simulink model "kalman_filter"  (R2021a)
settings: Solver=FixedStepAuto  StartTime=0.0  StopTime=30-0.2  FixedStep=dt  RelTol=1e-3
values from neighbouring files (symbols this model uses):
  dt = 0.2    [kalman_filter_data.mat]
  m = 1000    [kalman_filter_data.mat]
  P = [1  0; 0  1]    [kalman_filter_data.mat]
  Q = [0.3  0; 0  0.1]    [kalman_filter_data.mat]
  r = 0.2    [kalman_filter_data.mat]
  R = 20    [kalman_filter_data.mat]
  x_hat = [0 0]    [kalman_filter_data.mat]
settings Model: Creator=Sıla The Magnificent  LastModifiedBy=Sıla The Magnificent

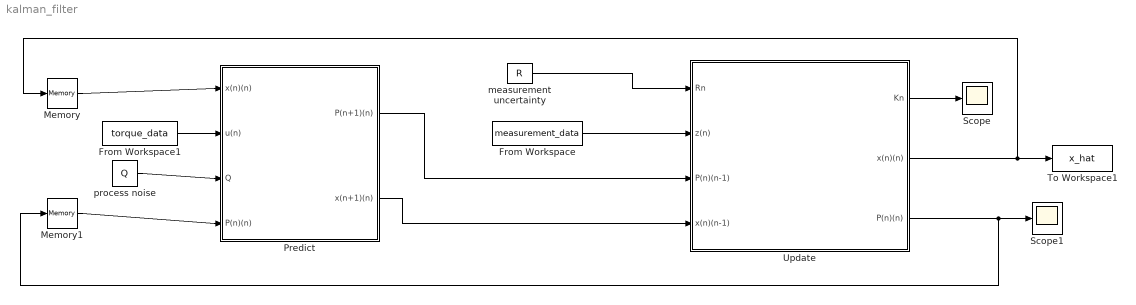
== system kalman_filter ==
  From Workspace : FromWorkspace  VariableName=measurement_data  SampleTime=dt
  From Workspace1 : FromWorkspace  VariableName=torque_data  SampleTime=dt
  Memory : Memory  InitialCondition=x_hat
  Memory1 : Memory  InitialCondition=P
  Predict : Subsystem
  Scope : Scope
  Scope1 : Scope
  To Workspace1 : ToWorkspace  VariableName=x_hat  SaveFormat=Timeseries  SampleTime=dt
  Update : Subsystem
  measurement uncertainty : Constant  Value=R  SampleTime=dt
  process noise : Constant  Value=Q  VectorParams1D=off  SampleTime=dt
  wires:
  From Workspace1/1 -> Predict/2(u(n))
  process noise/1 -> Predict/3(Q)
  measurement uncertainty/1 -> Update/1(Rn)
  From Workspace/1 -> Update/2(z(n))
  Predict/2(x(n+1)(n)) -> Update/4(x(n)(n-1))
  Predict/1(P(n+1)(n)) -> Update/3(P(n)(n-1))
  Update/1(Kn) -> Scope/1
  Update/2(x(n)(n)) -> Memory/1, To Workspace1/1
  Update/3(P(n)(n)) -> Scope1/1, Memory1/1
  Memory/1 -> Predict/1(x(n)(n))
  Memory1/1 -> Predict/4(P(n)(n))

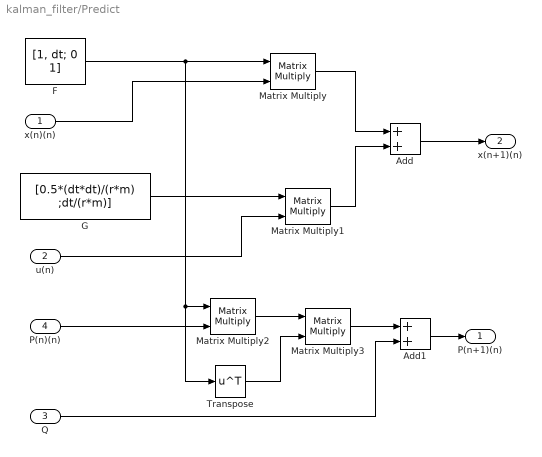
== system kalman_filter/Predict ==
  x(n)(n) : Inport
  u(n) : Inport  Port=2
  Q : Inport  Port=3
  P(n)(n) : Inport  Port=4
  Add : Sum
  Add1 : Sum
  F : Constant  Value=[1, dt; 0 1]  VectorParams1D=off  SampleTime=dt
  G : Constant  Value=[0.5*(dt*dt)/(r*m) ;dt/(r*m)]  VectorParams1D=off  SampleTime=dt
  Matrix Multiply{,1..3} (4 alike) : Product  Multiplication=Matrix(*)
  Transpose : Math  Operator=transpose  SaturateOnIntegerOverflow=on
  P(n+1)(n) : Outport
  x(n+1)(n) : Outport  Port=2
  wires:
  F/1 -> Matrix Multiply/1, Matrix Multiply2/1, Transpose/1
  x(n)(n)/1 -> Matrix Multiply/2
  Matrix Multiply/1 -> Add/1
  G/1 -> Matrix Multiply1/1
  u(n)/1 -> Matrix Multiply1/2
  Matrix Multiply1/1 -> Add/2
  Add/1 -> x(n+1)(n)/1
  P(n)(n)/1 -> Matrix Multiply2/2
  Matrix Multiply2/1 -> Matrix Multiply3/1
  Transpose/1 -> Matrix Multiply3/2
  Matrix Multiply3/1 -> Add1/1
  Q/1 -> Add1/2
  Add1/1 -> P(n+1)(n)/1

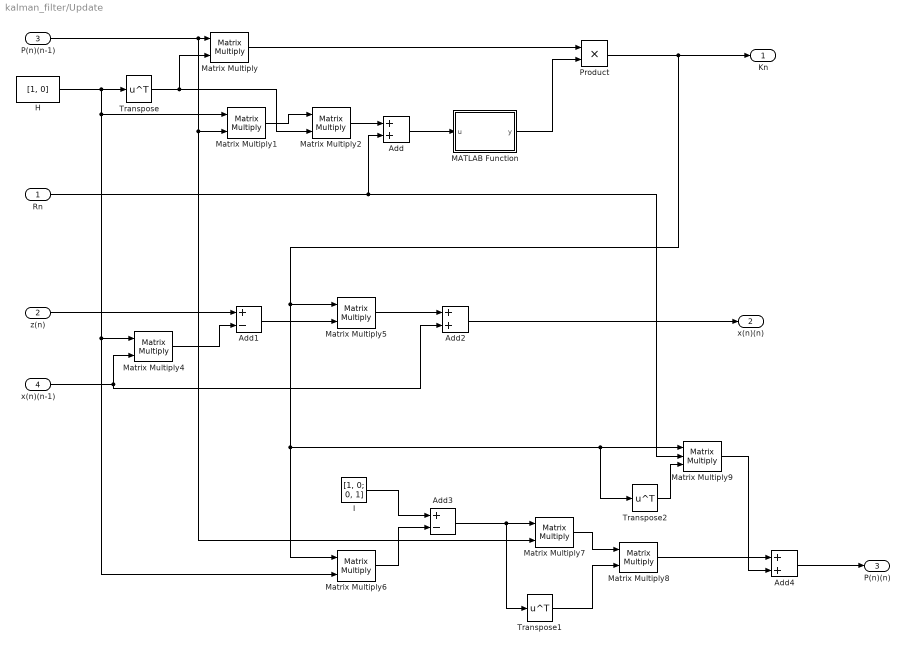
== system kalman_filter/Update ==
  Rn : Inport
  z(n) : Inport  Port=2
  P(n)(n-1) : Inport  Port=3
  x(n)(n-1) : Inport  Port=4
  Add : Sum
  Add1 : Sum  Inputs=+-
  Add2 : Sum
  Add3 : Sum  Inputs=+-
  Add4 : Sum
  H : Constant  Value=[1, 0]  VectorParams1D=off  SampleTime=dt
  I : Constant  Value=[1, 0; 0, 1]  VectorParams1D=off  SampleTime=dt
  MATLAB Function : MATLAB Function  TreatAsAtomicUnit=on
  Matrix Multiply{,1..2,4..8} (8 alike) : Product  Multiplication=Matrix(*)
  Matrix Multiply9 : Product  Inputs=3  Multiplication=Matrix(*)
  Product : Product
  Transpose : Math  Operator=transpose  SaturateOnIntegerOverflow=on
  Transpose1 : Math  Operator=transpose  SaturateOnIntegerOverflow=on
  Transpose2 : Math  Operator=transpose  SaturateOnIntegerOverflow=on
  Kn : Outport
  x(n)(n) : Outport  Port=2
  P(n)(n) : Outport  Port=3
  wires:
  H/1 -> Matrix Multiply6/2, Matrix Multiply4/1, Matrix Multiply1/1, Transpose/1
  P(n)(n-1)/1 -> Matrix Multiply1/2, Matrix Multiply7/2, Matrix Multiply/1
  Transpose/1 -> Matrix Multiply2/2, Matrix Multiply/2
  Matrix Multiply1/1 -> Matrix Multiply2/1
  Matrix Multiply2/1 -> Add/1
  Add/1 -> MATLAB Function/1(u)
  Matrix Multiply/1 -> Product/1
  Product/1 -> Matrix Multiply5/1, Matrix Multiply6/1, Transpose2/1, Matrix Multiply9/1, Kn/1
  x(n)(n-1)/1 -> Add2/2, Matrix Multiply4/2
  Matrix Multiply4/1 -> Add1/2
  z(n)/1 -> Add1/1
  Add1/1 -> Matrix Multiply5/2
  Matrix Multiply5/1 -> Add2/1
  Add2/1 -> x(n)(n)/1
  I/1 -> Add3/1
  Matrix Multiply6/1 -> Add3/2
  Add3/1 -> Transpose1/1, Matrix Multiply7/1
  Matrix Multiply7/1 -> Matrix Multiply8/1
  Transpose1/1 -> Matrix Multiply8/2
  Matrix Multiply8/1 -> Add4/1
  Rn/1 -> Add/2, Matrix Multiply9/2
  Transpose2/1 -> Matrix Multiply9/3
  Matrix Multiply9/1 -> Add4/2
  Add4/1 -> P(n)(n)/1
  MATLAB Function/1(y) -> Product/2

== matlab function kalman_filter/Update/MATLAB Function ==
  data: u input; y output
function y = inverseMatrix(u)
    y = inv(u);
end
